simulink model "timeresponse"  (R2023b)
settings: Solver=VariableStepAuto  StartTime=0.0  StopTime=10.0  RelTol=1e-3
libraries: audiosources x2, matrix_library x2, dspsnks4 x1
settings Model: Creator=Thinkpad  LastModifiedBy=Thinkpad

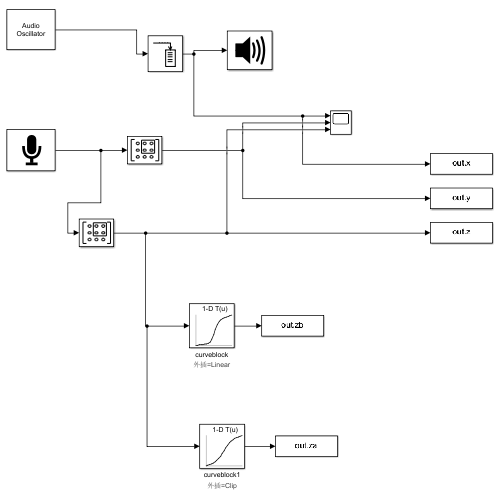
[thumbnail: Simulink's stored preview of the top-level diagram]
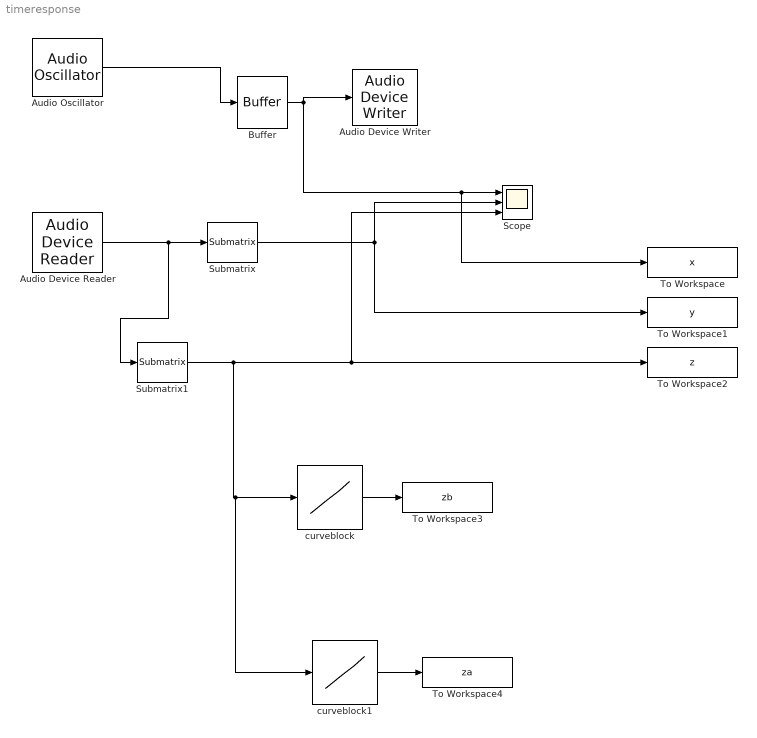
== system timeresponse ==
  Audio Device Reader : audiosources/Audio Device Reader  Driver=DirectSound  Device=Default  SampleRate=48000  NumChannels=2  SamplesPerFrame=1024  BitDepth=16-bit integer  NumBuffers=10  DefaultInputChannelMapping=on  InputChannelMapping=1:2  OutputNumOverrunSamples=off  OutputDataType=double  DriverIdx=1  DeviceWarnFlag=麦克风 (Scarlett 2i2 USB)
  Audio Device Writer : dspsnks4/Audio Device Writer  Driver=DirectSound  Device=Default  InheritSampleRate=on  SampleRate=44100  BitDepth=16-bit integer  BufferSize=4096  NumBuffers=10  DefaultOutputChannelMapping=on  OutputChannelMapping=1:2  OutputNumUnderrunSamples=off  DriverIdx=1  DeviceWarnFlag=扬声器 (Scarlett 2i2 USB)
  Audio Oscillator : audiosources/Audio Oscillator  FrequencyPort=off  Frequency=100  AmplitudePort=off  Amplitude=1  DCOffsetPort=off  PhaseOffset=0  DCOffset=0  WidthPort=off  Width=1  DutyCyclePort=off  DutyCycle=0.5  SampsPerFrame=1024  Fs=48000  OutputDataType=double  SimulateUsing=Code generation
      settings: SignalType=sine
  Buffer : Buffer  N=1024  OutputFrames=off
  Scope : Scope  NumInputPorts=3
  Submatrix : matrix_library/Submatrix  RowSpan=All rows  RowStartMode=First  RowStartIndex=1  RowEndMode=Last  RowEndIndex=1  ColSpan=One column  ColStartMode=First  ColStartIndex=1  ColEndMode=Last  ColEndIndex=1
  Submatrix1 : matrix_library/Submatrix  RowSpan=All rows  RowStartMode=First  RowStartIndex=1  RowEndMode=Last  RowEndIndex=1  ColSpan=One column  ColStartMode=Last  ColStartIndex=1  ColEndMode=Last  ColEndIndex=1
  To Workspace : ToWorkspace  VariableName=x  SampleTime=-1
      settings: Save2DSignal=2-D array (concatenate along first dimension)
  To Workspace1 : ToWorkspace  VariableName=y  SampleTime=-1
      settings: Save2DSignal=2-D array (concatenate along first dimension)
  To Workspace2 : ToWorkspace  VariableName=z  SampleTime=-1
      settings: Save2DSignal=2-D array (concatenate along first dimension)
  To Workspace3 : ToWorkspace  VariableName=zb  SampleTime=-1
      settings: Save2DSignal=2-D array (concatenate along first dimension)
  To Workspace4 : ToWorkspace  VariableName=za  SampleTime=-1
      settings: Save2DSignal=2-D array (concatenate along first dimension)
  curveblock : Lookup_n-D  NumberOfTableDimensions=1  LookupTableObject=curveBlockParameters  BreakpointsForDimension1=[-1;-0.9;-0.8;-0.7;-0.6;-0.5;-0.4;-0.3;-0.2;-0.1;0;0.1;0.2;0.3;0.4;0.5;0.6;0.7;0.8;0.9;1]  IndexSearchMethod=Evenly spaced points  Table=[-0.167560042983267;-0.164025163142684;-0.161081341613373;-0.1581299121418;-0.155070428348124;-0.151567098992156;-0.147238873839992;-0.140027808357011;-0.124302137029194;-0.0920389285159472;-0.0401939231670865;0.0229546619907531;0.0790180810327095;0.115927986026895;0.136076263194191;0.149169450966101;0.159450399835154;0.16858260358024;0.176944662952015;0.184016831341936;0.193011872253637]  RemoveProtectionInput=on  InternalRulePriority=Speed  RndMeth=Simplest
      settings: AttributesFormatString=外插=%<ExtrapMethod>
  curveblock1 : Lookup_n-D  NumberOfTableDimensions=1  LookupTableObject=curveBlockParameters  BreakpointsForDimension1=[-1;-0.9;-0.8;-0.7;-0.6;-0.5;-0.4;-0.3;-0.2;-0.1;0;0.1;0.2;0.3;0.4;0.5;0.6;0.7;0.8;0.9;1]  IndexSearchMethod=Evenly spaced points  Table=[-0.364415394102135;-0.343279098400792;-0.325914785320255;-0.309461387648919;-0.29101180324297;-0.268653413826881;-0.23705456393864;-0.190454015492191;-0.130630740764401;-0.0651564645099696;-0.000535625153878212;0.0641378054282629;0.129741738878902;0.189737863498686;0.236520373839183;0.268282074158697;0.290889331383481;0.310190052697053;0.328545148391925;0.346881716916853;0.366415718641209]  ExtrapMethod=Clip  RemoveProtectionInput=on  InternalRulePriority=Speed  RndMeth=Simplest
      settings: AttributesFormatString=外插=%<ExtrapMethod>
  wires:
  Audio Device Reader/1 -> Submatrix1/1, Submatrix/1
  Submatrix/1 -> Scope/2, To Workspace1/1
  Audio Oscillator/1 -> Buffer/1
  Buffer/1 -> Audio Device Writer/1, To Workspace/1, Scope/1
  Submatrix1/1 -> curveblock1/1, curveblock/1, Scope/3, To Workspace2/1
  curveblock/1 -> To Workspace3/1
  curveblock1/1 -> To Workspace4/1
